simulink model "CAN_test"  (R2016b)
settings: Solver=FixedStepDiscrete  StartTime=0.0  StopTime=100  FixedStep=0.001  RelTol=1e-3  EnableMultiTasking=on
values from neighbouring files (symbols this model uses):
  x2 = 340    [data_trigger.m]    (also in normalize.m = d(t(3):t(4),1); normalizeV2.m = d(t(3):t(4),1))
undefined symbols (not defined in the file or in its folder): bit, Standard
libraries: slrtsoftinglib x5, canmsglib x4, slrtlib x1
settings Model: xpc_rtwmakecfg_data=_xpccanac2pci_  SimulationMode=external  Creator=Administrator  LastModifiedBy=1108gotthem
settings SolverCC: EnableConcurrentExecution=on  ConcurrentTasks=on
settings DataIOCC: LimitDataPoints=on  SaveFormat=Array  SignalLoggingSaveFormat=ModelDataLogs  SaveOutput=off  SignalLogging=off  DSMLogging=off  SaveTime=off
settings OptimizationCC: OptimizeBlockIOStorage=off  BufferReuse=off  GlobalBufferReuse=off  ExpressionFolding=off  ExpressionDepthLimit=2147483647  LocalBlockOutputs=off  EfficientFloat2IntCast=on  SimCompilerOptimization=on
settings DebuggingCC: UnderspecifiedInitializationDetection=Classic  MergeDetectMultiDrivingBlocksExec=none  SolverPrmCheckMsg=warning  FcnCallInpInsideContextMsg=warning  StateNameClashWarn=warning  SFUnexpectedBacktrackingDiag=warning  SFNoUnconditionalDefaultTransitionDiag=warning  SFExecutionAtInitializationDiag=none
settings HardwareCC: ProdBitPerPointer=32  ProdBitPerSizeT=32  ProdBitPerPtrDiffT=32  ProdLargestAtomicFloat=None  ProdWordSize=32  ProdLongLongMode=on  ProdHWDeviceType=Generic->32-bit x86 compatible
settings ModelReferenceCC: PropagateSignalLabelsOutOfModel=off
settings RTWCC: SystemTargetFile=slrt.tlc  TemplateMakefile=slrt_default_tmf  Description=Simulink Real-Time  RTWVerbose=off  RTWCompilerOptimization=on
settings CodeAppCC: GenerateComments=off  SimulinkBlockComments=off
settings SimulinkRealTimeCC: RL32LogBufSizeModifier=100  xpcDblBuff=on  xPCConcurrentTasks=on
settings ConfigComp: CovMetricSettings=dw  CovHtmlReporting=on  CovSaveCumulativeToWorkspaceVar=on  CovSaveSingleToWorkspaceVar=on  CovExternalEMLEnable=off

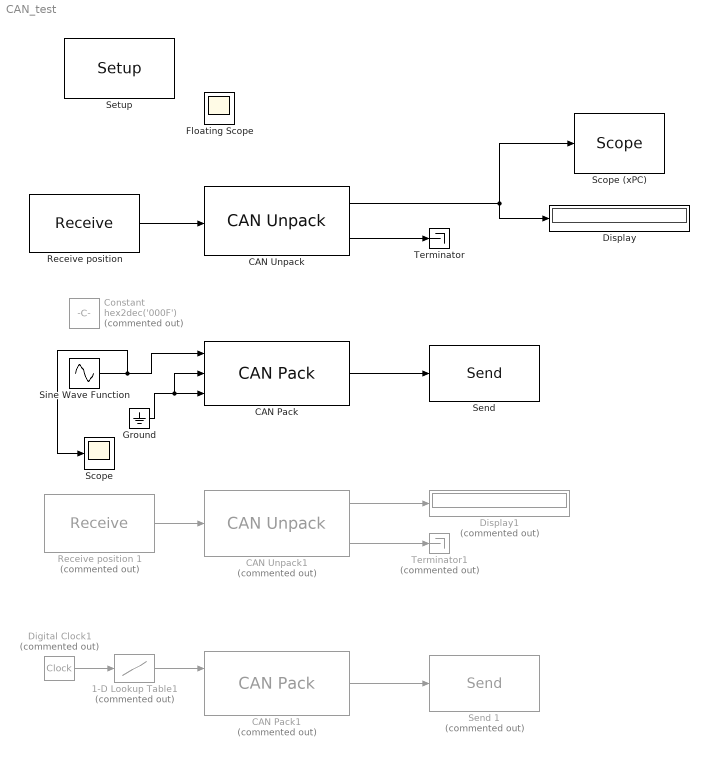
== system CAN_test ==
  1-D Lookup Table1 : Lookup_n-D  Commented=on  NumberOfTableDimensions=1  BreakpointsForDimension1=t  Table=x2  InterpMethod=Cubic spline  ExtrapMethod=Clip  RndMeth=Simplest  InputSameDT=on
  CAN Pack : canmsglib/CAN Pack  MsgList=(none)  MsgName=CAN Msg  MsgIDType=Standard (11-bit identifier)  MsgIdentifier=hex2dec('201')  MsgLength=8  SignalInfo=current$0$16$1$1$1$0$1$0$-Inf$Inf$#null$16$16$1$1$1$0$1$0$-Inf$Inf$#null2$32$32$1$1$1$0$1$0$-Inf$Inf$#  NSignals=3  StartBits=str2num('[int32(0);int32(16);int32(32)]')  SignalSizes=str2num('[int32(16);int32(16);int32(32)]')  ByteOrders=str2num('[int32(1);int32(1);int32(1)]')  DataTypes=str2num('[int32(1);int32(1);int32(1)]')  MultiplexTypes=str2num('[int32(1);int32(1);int32(1)]')  MultiplexValues=str2num('[double(0);double(0);double(0)]')  Factors=str2num('[double(1);double(1);double(1)]')  Offsets=str2num('[double(0);double(0);double(0)]')  Minimums=str2num('[double(-Inf);double(-Inf);double(-Inf)]')  Maximums=str2num('[double(Inf);double(Inf);double(Inf)]')  Remote=off
      settings: DataFormat=manually specified signals
  CAN Pack1 : canmsglib/CAN Pack  Commented=on  MsgList=(none)  MsgName=CAN Msg  MsgIDType=Standard (11-bit identifier)  MsgIdentifier=hex2dec('302')  MsgLength=8  SignalInfo=position$0$32$1$1$1$0$1$0$-Inf$Inf$#velocity$32$32$1$1$1$0$1$0$-Inf$Inf$#  NSignals=2  StartBits=str2num('[int32(0);int32(32)]')  SignalSizes=str2num('[int32(32);int32(32)]')  ByteOrders=str2num('[int32(1);int32(1)]')  DataTypes=str2num('[int32(1);int32(1)]')  MultiplexTypes=str2num('[int32(1);int32(1)]')  MultiplexValues=str2num('[double(0);double(0)]')  Factors=str2num('[double(1);double(1)]')  Offsets=str2num('[double(0);double(0)]')  Minimums=str2num('[double(-Inf);double(-Inf)]')  Maximums=str2num('[double(Inf);double(Inf)]')  Remote=off
      settings: DataFormat=manually specified signals
  CAN Unpack : canmsglib/CAN Unpack  MsgList=(none)  MsgName=CAN Msg  MsgIDType=Standard (11-bit identifier)  MsgIdentifier=hex2dec('181')  MsgLength=8  SignalInfo=position$0$32$1$1$1$0$1$0$-Inf$Inf$#null$32$32$1$2$1$0$1$0$-Inf$Inf$#  NSignals=2  IDPort=off  TimestampPort=off  ErrorPort=off  RemotePort=off  LengthPort=off  StatusPort=off  StartBits=str2num('[int32(0);int32(32)]')  SignalSizes=str2num('[int32(32);int32(32)]')  ByteOrders=str2num('[int32(1);int32(1)]')  DataTypes=str2num('[int32(1);int32(2)]')  MultiplexTypes=str2num('[int32(1);int32(1)]')  MultiplexValues=str2num('[double(0);double(0)]')  Factors=str2num('[double(1);double(1)]')  Offsets=str2num('[double(0);double(0)]')  Minimums=str2num('[double(-Inf);double(-Inf)]')  Maximums=str2num('[double(Inf);double(Inf)]')
  CAN Unpack1 : canmsglib/CAN Unpack  Commented=on  MsgList=(none)  MsgName=CAN Msg  MsgIDType=Standard (11-bit identifier)  MsgIdentifier=hex2dec('382')  MsgLength=8  SignalInfo=Statusword$0$16$1$2$1$0$1$0$-Inf$Inf$#Position$16$32$1$1$1$0$1$0$-Inf$Inf$#null$48$16$1$2$1$0$1$0$-Inf$Inf$#  NSignals=3  IDPort=off  TimestampPort=off  ErrorPort=off  RemotePort=off  LengthPort=off  StatusPort=off  StartBits=str2num('[int32(0);int32(16);int32(48)]')  SignalSizes=str2num('[int32(16);int32(32);int32(16)]')  ByteOrders=str2num('[int32(1);int32(1);int32(1)]')  DataTypes=str2num('[int32(2);int32(1);int32(2)]')  MultiplexTypes=str2num('[int32(1);int32(1);int32(1)]')  MultiplexValues=str2num('[double(0);double(0);double(0)]')  Factors=str2num('[double(1);double(1);double(1)]')  Offsets=str2num('[double(0);double(0);double(0)]')  Minimums=str2num('[double(-Inf);double(-Inf);double(-Inf)]')  Maximums=str2num('[double(Inf);double(Inf);double(Inf)]')
  Constant : Constant  Commented=on  Value=hex2dec('000F')
  Digital Clock1 : DigitalClock  Commented=on  SampleTime=0.001
  Display : Display
      settings: Format=hex (Stored Integer)
  Display1 : Display  Commented=on
      settings: Format=hex (Stored Integer)
  Ground : Ground
  "Receive position " : slrtsoftinglib/CAN-AC2-PCI SJA 1000/Receive   board=1  canPort=CAN 1  range=Standard (11-bit)  ids=hex2dec('181')  lengths=8  output=CAN_MESSAGE data type  inten=off  ts=0.001  ididx=[0]
  Receive position 1 : slrtsoftinglib/CAN-AC2-PCI SJA 1000/Receive   Commented=on  board=1  canPort=CAN 1  range=Standard (11-bit)  ids=hex2dec('382')  lengths=8  output=CAN_MESSAGE data type  inten=off  ts=0.001  ididx=[1]
  Scope : Scope
  "Scope (xPC) " : slrtlib/Displays and Logging/Scope   scopeno=1  scopetype=Target  autostart=on  viewmode=Graphical rolling  formatstr='%15.6f'  grid=on  ylimits=[-700,700]  nosamples=13001  noprepostsamples=0  interleave=1  triggermode=FreeRun  triggersignal=1  trigsignalfromport=off  triggerlevel=0.0  triggerslope=Either  triggerscope=1  triggersample=0  filename=data.dat  mode=Lazy  writesize=512  autorestart=off  dynamicfilemode=off  maxwritefilesize=512*1024^2
  "Send " : slrtsoftinglib/CAN-AC2-PCI SJA 1000/Send   board=1  canPort=CAN 1  range=Standard (11-bit)  ids=hex2dec('201')  sizes=8  output=off  ts=0.001  ididx=[1]
  Send 1 : slrtsoftinglib/CAN-AC2-PCI SJA 1000/Send   Commented=on  board=1  canPort=CAN 1  range=Standard (11-bit)  ids=hex2dec('302')  sizes=8  output=off  ts=0.001  ididx=[2]
  "Setup " : slrtsoftinglib/CAN-AC2-PCI SJA 1000/Setup   board=1  can1bus=Highspeed (ISO 11898)  can1Baudrate=1 MBaud  can1UserBR=[1,1,4,3]  can2bus=Highspeed (ISO 11898)  can2Baudrate=1 MBaud  can2UserBR=[1,1,4,3]  init=pdo_start  term=pdo_stop  bus_off_out=off  bus_off_rec=Off  ioBaseAddress=-1
  Sine Wave Function : Sin  Amplitude=600  SampleTime=.001
  Terminator : Terminator
  Terminator1 : Terminator  Commented=on
  Floating Scope : Scope
  wires:
  "Receive position "/1 -> CAN Unpack/1
  CAN Unpack/1 -> "Scope (xPC) "/1, Display/1
  CAN Pack/1 -> "Send "/1
  Ground/1 -> CAN Pack/2, CAN Pack/3
  Receive position 1/1 -> CAN Unpack1/1
  CAN Unpack1/1 -> Display1/1
  CAN Unpack1/3 -> Terminator1/1
  CAN Pack1/1 -> Send 1/1
  Digital Clock1/1 -> 1-D Lookup Table1/1
  1-D Lookup Table1/1 -> CAN Pack1/1
  CAN Unpack/2 -> Terminator/1
  Sine Wave Function/1 -> Scope/1, CAN Pack/1
